simulink model "check_ndtm_drive"  (R2018b)
settings: configuration reference "Physics" (kept outside this file)
settings Model: DataDictionary=check_ndtm.sldd  OrderedModelArguments=off  Creator=wischnewski  LastModifiedBy=ga25xiw

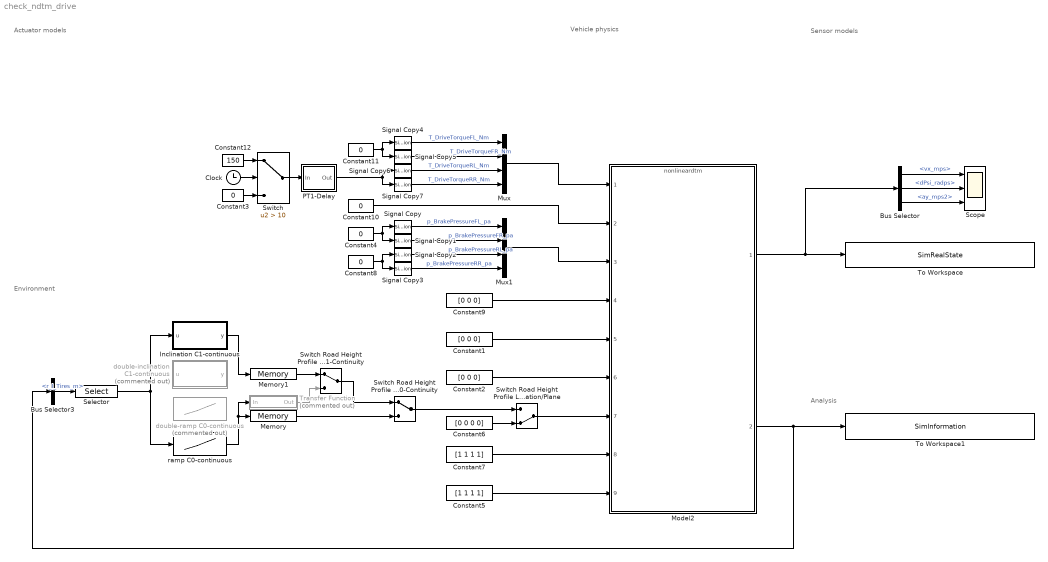
== system check_ndtm_drive ==
  note: Actuator models
  note: Vehicle physics
  note: Environment
  note: Analysis
  note: Sensor models
  Bus Selector : BusSelector  OutputSignals=vx_mps,dPsi_radps,ay_mps2
  Bus Selector3 : BusSelector  OutputSignals=Wheel.r_I_Tires_m
  Clock : Clock
  Constant1 : Constant  Value=[0 0 0]
  Constant{3..4,8,10..11} (5 alike) : Constant  Value=0
  Constant12 : Constant  Value=150
  Constant2 : Constant  Value=[0 0 0]
  Constant5 : Constant  Value=[1 1 1 1]
  Constant6 : Constant  Value=[0 0 0 0]
  Constant7 : Constant  Value=[1 1 1 1]
  Constant9 : Constant  Value=[0 0 0]
  Inclination C1-continuous : MATLAB Function  TreatAsAtomicUnit=on
  Memory : Memory
  Memory1 : Memory
  Model2 : ModelReference  ModelNameDialog=nonlineardtm  ParameterArgumentNames=x0_initialstates  ParameterArgumentValues=[0 0 0 0 0 -pi/2]  UsingDefaultArgumentValue=0  SimulationMode=Normal  ModelReferenceVersion=1.712
  Mux : Mux
  Mux1 : Mux
  PT1-Delay : Subsystem
  Scope : Scope  NumInputPorts=3
  Selector : Selector  NumberOfDimensions=2  InputPortWidth=3  IndexOptions=Index vector (dialog),Select all  Indices=1,1  OutputSizes=1,1
  Signal Copy{,1..7} (8 alike) : SignalConversion  OverrideOpt=off
  Switch : Switch  Criteria=u2 > Threshold  Threshold=10
  Switch Road Height Profile C1-Continuity/C0-Continuity : ManualSwitch
  Switch Road Height Profile C1-Continuity/Pseudo-C1-Continuity : ManualSwitch
  Switch Road Height Profile Longitudinal Inclination/Plane : ManualSwitch  CurrentSetting=0
  To Workspace : ToWorkspace  VariableName=SimRealState  SaveFormat=Timeseries  SampleTime=-1
  To Workspace1 : ToWorkspace  VariableName=SimInformation  SaveFormat=Timeseries  SampleTime=-1
  Transfer Function : Subsystem  Commented=on
  double-inclination C1-continuous : MATLAB Function  Commented=on  TreatAsAtomicUnit=on
  double-ramp C0-continuous : Lookup_n-D  Commented=on  NumberOfTableDimensions=1  BreakpointsForDimension1=[0 100 500 700 1100 2000]  Table=[0 0 -20 -20 0 0]  InternalRulePriority=Speed  RndMeth=Simplest  InputSameDT=on
  ramp C0-continuous : Lookup_n-D  NumberOfTableDimensions=1  BreakpointsForDimension1=[0 100 500 1000]  Table=[0 0 -20 -20]  InternalRulePriority=Speed  RndMeth=Simplest  InputSameDT=on
  wires:
  Constant4/1 -> Signal Copy1/1, Signal Copy/1
  Bus Selector/1 -> Scope/1  "<vx_mps>"
  Bus Selector/2 -> Scope/2  "<dPsi_radps>"
  Bus Selector/3 -> Scope/3  "<ay_mps2>"
  Model2/1 -> Bus Selector/1, To Workspace/1
  Constant9/1 -> Model2/4
  Constant1/1 -> Model2/5
  Constant2/1 -> Model2/6
  Constant7/1 -> Model2/8
  Constant5/1 -> Model2/9
  Bus Selector3/1 -> Selector/1  "<r_I_Tires_m>"
  Constant6/1 -> Switch Road Height Profile Longitudinal Inclination/Plane/2
  Model2/2 -> To Workspace1/1, Bus Selector3/1
  Switch Road Height Profile Longitudinal Inclination/Plane/1 -> Model2/7
  Selector/1 -> ramp C0-continuous/1, Inclination C1-continuous/1(u)
  Clock/1 -> Switch/2
  Constant3/1 -> Switch/3
  Constant12/1 -> Switch/1
  Switch/1 -> PT1-Delay/1(In)
  Switch Road Height Profile C1-Continuity/C0-Continuity/1 -> Switch Road Height Profile Longitudinal Inclination/Plane/1
  ramp C0-continuous/1 -> Transfer Function/1(In), Memory/1
  Inclination C1-continuous/1(y) -> Memory1/1
  Transfer Function/1(Out) -> Switch Road Height Profile C1-Continuity/Pseudo-C1-Continuity/2
  Memory/1 -> Switch Road Height Profile C1-Continuity/C0-Continuity/2
  Switch Road Height Profile C1-Continuity/Pseudo-C1-Continuity/1 -> Switch Road Height Profile C1-Continuity/C0-Continuity/1
  Memory1/1 -> Switch Road Height Profile C1-Continuity/Pseudo-C1-Continuity/1
  Signal Copy/1 -> Mux1/1  "p_BrakePressureFL_pa"
  Signal Copy1/1 -> Mux1/2  "p_BrakePressureFR_pa"
  Signal Copy2/1 -> Mux1/3  "p_BrakePressureRL_pa"
  Signal Copy3/1 -> Mux1/4  "p_BrakePressureRR_pa"
  Constant8/1 -> Signal Copy3/1, Signal Copy2/1
  PT1-Delay/1(Out) -> Signal Copy6/1, Signal Copy7/1
  Signal Copy7/1 -> Mux/4  "T_DriveTorqueRR_Nm"
  Signal Copy6/1 -> Mux/3  "T_DriveTorqueRL_Nm"
  Signal Copy5/1 -> Mux/2  "T_DriveTorqueFR_Nm"
  Signal Copy4/1 -> Mux/1  "T_DriveTorqueFL_Nm"
  Constant11/1 -> Signal Copy4/1, Signal Copy5/1
  Constant10/1 -> Model2/2
  Mux1/1 -> Model2/3
  Mux/1 -> Model2/1

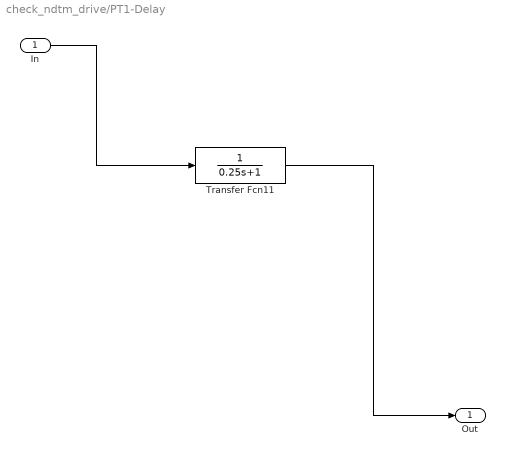
== system check_ndtm_drive/PT1-Delay ==
  In : Inport
  Transfer Fcn11 : TransferFcn  Denominator=[0.25 1]
  Out : Outport
  wires:
  In/1 -> Transfer Fcn11/1
  Transfer Fcn11/1 -> Out/1

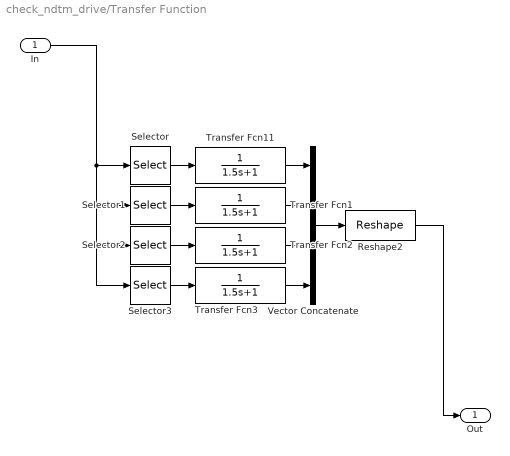
== system check_ndtm_drive/Transfer Function ==
  In : Inport
  Reshape2 : Reshape  OutputDimensionality=Row vector (2-D)
  Selector : Selector  NumberOfDimensions=2  InputPortWidth=12  IndexOptions=Index vector (dialog),Index vector (dialog)  Indices=[1],1  OutputSizes=1,1
  Selector1 : Selector  NumberOfDimensions=2  InputPortWidth=12  IndexOptions=Index vector (dialog),Index vector (dialog)  Indices=1,2  OutputSizes=1,1
  Selector2 : Selector  NumberOfDimensions=2  InputPortWidth=12  IndexOptions=Index vector (dialog),Index vector (dialog)  Indices=1,3  OutputSizes=1,1
  Selector3 : Selector  NumberOfDimensions=2  InputPortWidth=12  IndexOptions=Index vector (dialog),Index vector (dialog)  Indices=1,3  OutputSizes=1,1
  Transfer Fcn{1..3,11} (4 alike) : TransferFcn  Denominator=[1.5 1]
  Vector Concatenate : Concatenate  NumInputs=4
  Out : Outport
  wires:
  Transfer Fcn3/1 -> Vector Concatenate/4
  Selector3/1 -> Transfer Fcn3/1
  Transfer Fcn2/1 -> Vector Concatenate/3
  Reshape2/1 -> Out/1
  In/1 -> Selector/1, Selector1/1, Selector2/1, Selector3/1
  Selector/1 -> Transfer Fcn11/1
  Selector2/1 -> Transfer Fcn2/1
  Selector1/1 -> Transfer Fcn1/1
  Transfer Fcn11/1 -> Vector Concatenate/1
  Transfer Fcn1/1 -> Vector Concatenate/2
  Vector Concatenate/1 -> Reshape2/1

== matlab function check_ndtm_drive/Inclination C1-continuous ==
  data: u input; y output
function y = fcn(u)

profil=zeros(1,4);

for i=1:4

if u(i)<=100
    profil(i)=0;
elseif u(i)>100 && u(i)<500
    profil(i)=-10-10*sin(pi/400*(u(i)-300));
elseif u(i)>=500
    profil(i)=-20;    
end    

y=profil;

end

== matlab function check_ndtm_drive/double-inclination C1-continuous ==
  data: u input; y output
function y = fcn(u)

profil=zeros(1,4);

for i=1:4
    
if u(i)>100 && u(i)<500
    profil(i)=-10-10*sin(pi/400*(u(i)-300));
elseif u(i)>=500 && u(i)<=700
    profil(i)=-20;
elseif u(i)>700 && u(i)<1100
    profil(i)=-10+10*sin(pi/400*(u(i)-900));
else
    profil(i)=0;
    
end    

y=profil;

end
